simulink model "OFDM_Tx_HW_bk"  (R2020a)
settings: Solver=FixedStepDiscrete  StartTime=0.0  StopTime=inf  RelTol=1e-3
InitFcn:
  | % Set parameters
  | fs = 1e6;
  | 
  | % Load all required variables
  | load('variables/read_addr_data');
  | load('variables/read_addr_cp');
  | load('variables/read_addr_pream');
  | load('variables/read_addr_rx');
  | load('variables/pilot');
  | load('variables/sc_index');
  | load('variables/LTSfreq');
  | load('variables/STSfreq');
  | load('variables/LTSread');
  | load('variables/STSread');
  | 
  | run ./scripts/rfgen;
values from neighbouring files (symbols this model uses):
  interpolation_single = dsp.SampleRateConverter('InputSampleRate', 1e6,     'OutputSampleRate', 256e6,     'Bandwidth', 812.5e3,     'OutputRateTolerance', 0,     'StopbandAttenuation', 100)    [filter_design_1mhz.m]
undefined symbols (not defined in the file or in its folder): CIC_fine_Rx, Interpolate, lib_interpolatetx, lib_ofdmtx, LTSfreq, LTSread, OFDMTx, pilot, read_addr_cp, read_addr_data, read_addr_pream, STSfreq, STSread
libraries: hdlsllib x47, xbsIndex_r4 x22, simulink x19, dspsigops x5, dspmlti4 x3, lib_ofdmrx x1, lib_rfsignalgenerator x1, dsphdlxfrm x1, dspobslib x1
(part 1 of 2)
settings Model: Creator=njb13206  LastModifiedBy=david
settings OptimizationCC: BlockReduction=off  ConditionallyExecuteInputs=off  DefaultParameterBehavior=Inlined
settings DebuggingCC: AlgebraicLoopMsg=error  IntegerOverflowMsg=none  ParameterPrecisionLossMsg=none  IntegerSaturationMsg=none
settings HardwareCC: ProdBitPerPointer=32  ProdBitPerSizeT=32  ProdBitPerPtrDiffT=32  ProdLargestAtomicFloat=None  ProdIntDivRoundTo=Undefined  ProdEndianess=Unspecified  ProdWordSize=32  ProdHWDeviceType=ASIC/FPGA->ASIC/FPGA  TargetBitPerPointer=64  TargetBitPerSizeT=64  TargetBitPerPtrDiffT=64  TargetLongLongMode=on  TargetIntDivRoundTo=Zero  TargetEndianess=LittleEndian  TargetWordSize=64  TargetHWDeviceType=Custom Processor->MATLAB Host Computer  ProdEqTarget=off

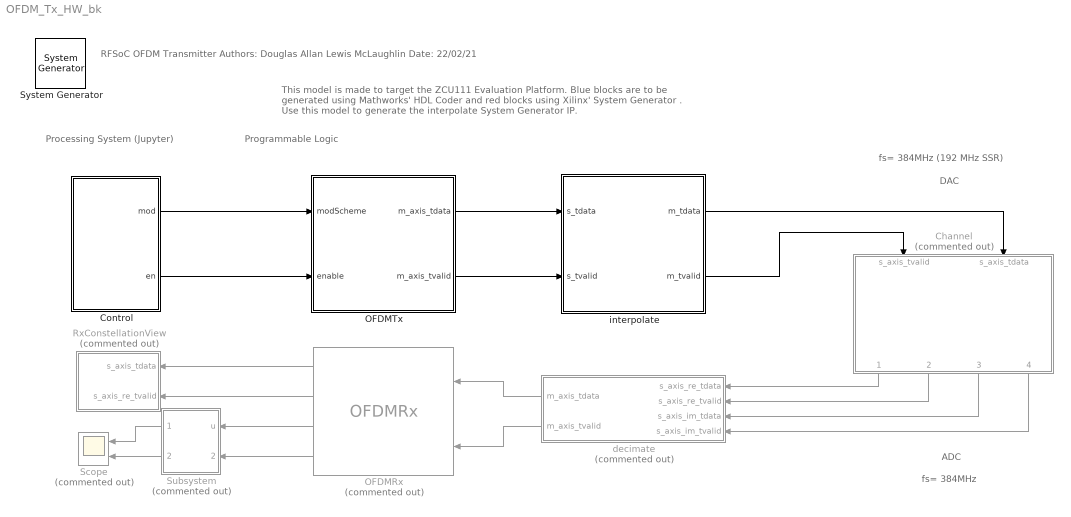
== system OFDM_Tx_HW_bk ==
  note: This model is made to target the ZCU111 Evaluation Platform. Blue blocks are to be generated using Mathworks' HDL Coder and red blocks using Xilinx' System Generator .
      |
      | Use this model to generate the interpolate System Generator IP.
  note: Programmable Logic
  note: Processing System (Jupyter)
  note: DAC
  note: fs= 384MHz (192 MHz SSR)
  note: ADC
  note: fs= 384MHz
  note: RFSoC OFDM Transmitter
      | Authors: Douglas Allan
      | Lewis McLaughlin
      | Date: 22/02/21
  " System Generator" : xbsIndex_r4/ System Generator  Tag=genX  xilinxfamily=zynquplusRFSOC  part=xczu28dr  speed=-2-e  package=ffvg1517  synthesis_tool=Vivado  clock_wrapper=Clock Enables  directory=./netlist  proj_type=Vivado  Synth_file=Vivado Synthesis Defaults  Impl_file=Vivado Implementation Defaults  testbench=off  simulink_period=1/256e6  sysclk_period=(1/256e6)*1e9  dcm_input_clock_period=10  incr_netlist=off  trim_vbits=Everywhere in SubSystem  dbl_ovrd=According to Block Masks  core_generation=According to Block Masks  run_coregen=off  deprecated_control=off  eval_field=0  block_type=sysgen
  Channel : Subsystem  Commented=on
  Control : Subsystem  mask{mod_mask=512QAM, en=on}
      mask prompts: mod_mask "Modulation"; en "Enable"
      mask init:
      | % RF Signal Generator
      | if strcmpi(get_param(gcb, 'mod_mask'), 'BPSK')
      |     mod = 0;
      | elseif strcmpi(get_param(gcb, 'mod_mask'), 'QPSK')
      |     mod = 1;
      | elseif strcmpi(get_param(gcb, 'mod_mask'), '8PSK')
      |     mod = 2;
      | elseif strcmpi(get_param(gcb, 'mod_mask'), '16QAM')
      |     mod = 3;
      | elseif strcmpi(get_param(gcb, 'mod_mask'), '32QAM')
      |     mod = 4;
      | elseif strcmpi(get_param(gcb, 'mod_mask'), '64QAM')
      |     mod = 5;
      | elseif strcmpi(get_param(gcb, 'mod_mask'), '128QAM')
      |     mod = 6;
      | elseif strcmpi(get_param(gcb, 'mod_mask'), '256QAM')
      |     mod = 7;
      | elseif strcmpi(get_param(gcb, 'mod_mask'), '512QAM')
      |     mod = 8;
      | elseif strcmpi(get_param(gcb, 'mod_mask'), '1024QAM')
      |     mod = 9;
      | end
      mask TypeOptions mod_mask: BPSK | QPSK | 8PSK | 16QAM | 32QAM | 64QAM | 128QAM | 256QAM | 512QAM | 1024QAM
      mask DialogControl DescGroupVar Prompt: RF Signal Generator
      mask DialogControl DescTextVar Prompt: Exposes parameters the user can control from Jupyter when running on the target.
      mask DialogControl Container3 Prompt: Control
  OFDMRx : lib_ofdmrx/OFDMRx  Commented=on  SystemSampleTime=-1  Latency=0  AutoFrameSizeCalculation=off
  OFDMTx : Subsystem  AncestorBlock=lib_ofdmtx/OFDMTx  TreatAsAtomicUnit=on
  RxConstellationView : Subsystem  Commented=on
  Scope : Scope  Commented=on  NumInputPorts=2
  Subsystem : Subsystem  Commented=on
  decimate : Subsystem  Commented=on
  interpolate : Subsystem  AncestorBlock=lib_interpolatetx/Interpolate
  wires:
  interpolate/1(m_tdata) -> Channel/2(s_axis_tdata)
  OFDMTx/1(m_axis_tdata) -> interpolate/1(s_tdata)
  OFDMTx/2(m_axis_tvalid) -> interpolate/2(s_tvalid)
  interpolate/2(m_tvalid) -> Channel/1(s_axis_tvalid)
  Channel/4(m_axis_im_tvalid) -> decimate/4(s_axis_im_tvalid)
  OFDMRx/1 -> RxConstellationView/1(s_axis_tdata)
  OFDMRx/2 -> RxConstellationView/2(s_axis_re_tvalid)
  Channel/1(m00_axis_re_tdata) -> decimate/1(s_axis_re_tdata)
  Channel/2(m_axis_re_tvalid) -> decimate/2(s_axis_re_tvalid)
  Channel/3(m01_axis_im_tdata) -> decimate/3(s_axis_im_tdata)
  decimate/2(m_axis_tvalid) -> OFDMRx/2
  decimate/1(m_axis_tdata) -> OFDMRx/1
  Control/1(mod) -> OFDMTx/1(modScheme)
  Control/2(en) -> OFDMTx/2(enable)
  OFDMRx/3 -> Subsystem/1(u)
  OFDMRx/4 -> Subsystem/2(tvalid)
  Subsystem/2(Out2) -> Scope/2
  Subsystem/1(Out1) -> Scope/1

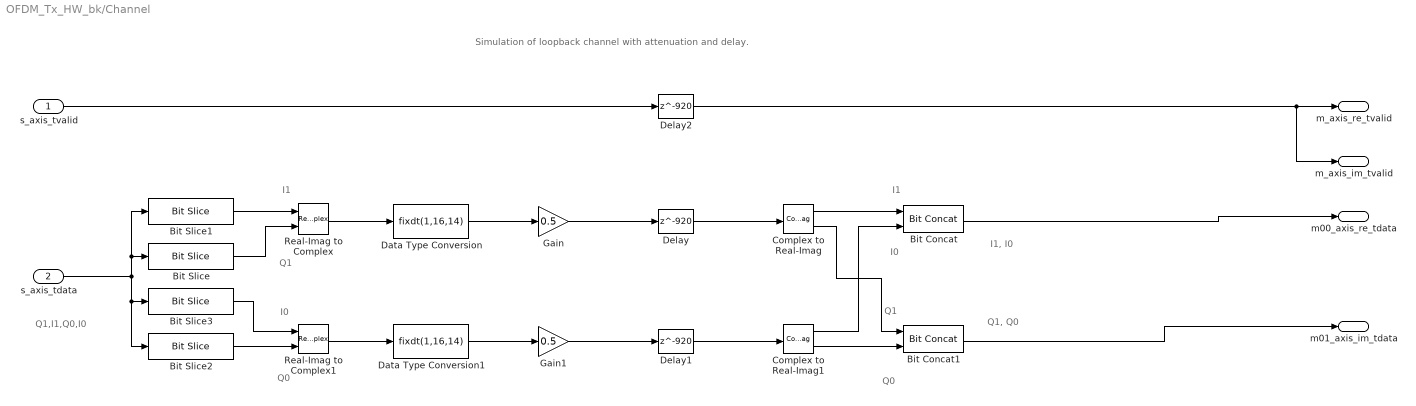
== system OFDM_Tx_HW_bk/Channel ==
  note: Q1, Q0
  note: I1, I0
  note: Q0
  note: I0
  note: Q1
  note: I1
  note: Q1,I1,Q0,I0
  note: Simulation of loopback channel with attenuation and delay.
  note: I1
  note: I0
  note: Q1
  note: Q0
  s_axis_tvalid : Inport
  s_axis_tdata : Inport  Port=2
  Bit Concat : hdlsllib/Logic and Bit Operations/Bit Concat  numInputs=2
  Bit Concat1 : hdlsllib/Logic and Bit Operations/Bit Concat  numInputs=2
  Bit Slice : hdlsllib/Logic and Bit Operations/Bit Slice  lidx=63  ridx=48
      settings: SourceProductBaseCode=SL
  Bit Slice1 : hdlsllib/Logic and Bit Operations/Bit Slice  lidx=47  ridx=32
      settings: SourceProductBaseCode=SL
  Bit Slice2 : hdlsllib/Logic and Bit Operations/Bit Slice  lidx=31  ridx=16
      settings: SourceProductBaseCode=SL
  Bit Slice3 : hdlsllib/Logic and Bit Operations/Bit Slice  lidx=15  ridx=0
      settings: SourceProductBaseCode=SL
  Complex to Real-Imag : ComplexToRealImag
  Complex to Real-Imag1 : ComplexToRealImag
  Data Type Conversion : DataTypeConversion  OutDataTypeStr=fixdt(1,16,14)  ConvertRealWorld=Stored Integer (SI)
  Data Type Conversion1 : DataTypeConversion  OutDataTypeStr=fixdt(1,16,14)  ConvertRealWorld=Stored Integer (SI)
  Delay : Delay  DelayLength=920
  Delay1 : Delay  DelayLength=920
  Delay2 : Delay  DelayLength=920
  Gain : Gain  Gain=0.5  ParamDataTypeStr=double  OutDataTypeStr=fixdt(1,16,14)
  Gain1 : Gain  Gain=0.5  ParamDataTypeStr=double  OutDataTypeStr=fixdt(1,16,14)
  Real-Imag to Complex : RealImagToComplex
  Real-Imag to Complex1 : RealImagToComplex
  m00_axis_re_tdata : Outport  VectorParamsAs1DForOutWhenUnconnected=off
  m_axis_re_tvalid : Outport  Port=2  VectorParamsAs1DForOutWhenUnconnected=off
  m01_axis_im_tdata : Outport  Port=3  VectorParamsAs1DForOutWhenUnconnected=off
  m_axis_im_tvalid : Outport  Port=4  VectorParamsAs1DForOutWhenUnconnected=off
  wires:
  Gain/1 -> Delay/1
  s_axis_tvalid/1 -> Delay2/1
  Delay/1 -> Complex to Real-Imag/1
  s_axis_tdata/1 -> Bit Slice1/1, Bit Slice/1, Bit Slice2/1, Bit Slice3/1
  Delay1/1 -> Complex to Real-Imag1/1
  Gain1/1 -> Delay1/1
  Bit Concat/1 -> m00_axis_re_tdata/1
  Bit Concat1/1 -> m01_axis_im_tdata/1
  Bit Slice/1 -> Real-Imag to Complex/2
  Bit Slice1/1 -> Real-Imag to Complex/1
  Bit Slice2/1 -> Real-Imag to Complex1/2
  Bit Slice3/1 -> Real-Imag to Complex1/1
  Real-Imag to Complex/1 -> Data Type Conversion/1
  Real-Imag to Complex1/1 -> Data Type Conversion1/1
  Complex to Real-Imag1/1 -> Bit Concat/2
  Complex to Real-Imag/1 -> Bit Concat/1
  Complex to Real-Imag1/2 -> Bit Concat1/2
  Complex to Real-Imag/2 -> Bit Concat1/1
  Data Type Conversion/1 -> Gain/1
  Data Type Conversion1/1 -> Gain1/1
  Delay2/1 -> m_axis_im_tvalid/1, m_axis_re_tvalid/1

== system OFDM_Tx_HW_bk/Control ==
  Constant2 : Constant  Value=en  OutDataTypeStr=boolean  SampleTime=1/(fs)
  Constant7 : Constant  Value=mod  VectorParams1D=off  OutDataTypeStr=uint32  SampleTime=1/(fs)
  Delay : Delay  DelayLength=randi(10)
  Delay3 : Delay  DelayLength=randi(10)
  mod : Outport  VectorParamsAs1DForOutWhenUnconnected=off
  en : Outport  Port=2  VectorParamsAs1DForOutWhenUnconnected=off
  wires:
  Constant2/1 -> Delay3/1
  Constant7/1 -> Delay/1
  Delay/1 -> mod/1
  Delay3/1 -> en/1

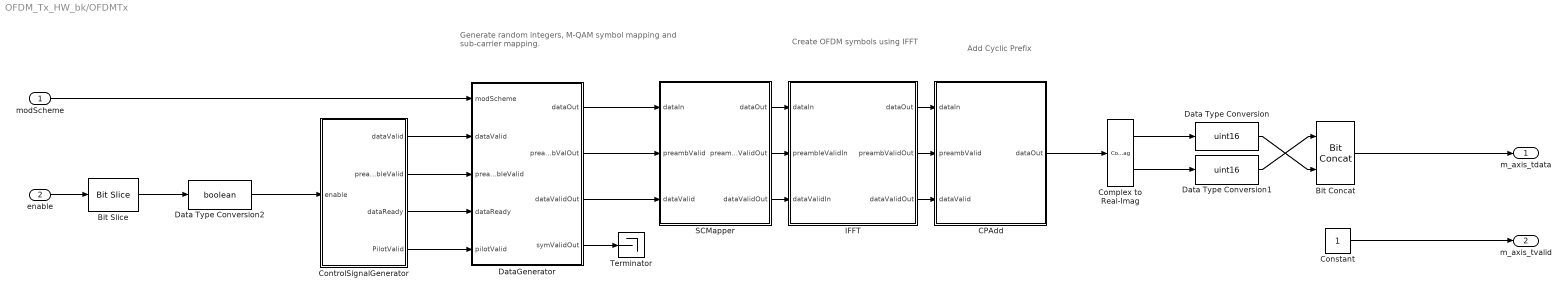
== system OFDM_Tx_HW_bk/OFDMTx ==
  note: Generate random integers, M-QAM symbol mapping and sub-carrier
      | mapping.
  note: Add Cyclic Prefix
  note: Create OFDM symbols using
      | IFFT
  modScheme : Inport
  enable : Inport  Port=2
  Bit Concat : hdlsllib/Logic and Bit Operations/Bit Concat  numInputs=2
  Bit Slice : hdlsllib/Logic and Bit Operations/Bit Slice  lidx=0  ridx=0
      settings: SourceProductBaseCode=SL
  CPAdd : Subsystem
  Complex to Real-Imag : ComplexToRealImag
  Constant : Constant  OutDataTypeStr=boolean  SampleTime=1/fs
  ControlSignalGenerator : Subsystem
  Data Type Conversion : DataTypeConversion  OutDataTypeStr=uint16  ConvertRealWorld=Stored Integer (SI)
  Data Type Conversion1 : DataTypeConversion  OutDataTypeStr=uint16  ConvertRealWorld=Stored Integer (SI)
  Data Type Conversion2 : DataTypeConversion  OutDataTypeStr=boolean  ConvertRealWorld=Stored Integer (SI)
  DataGenerator : Subsystem
  IFFT : Subsystem
  SCMapper : Subsystem
  Terminator : Terminator
  m_axis_tdata : Outport  VectorParamsAs1DForOutWhenUnconnected=off
  m_axis_tvalid : Outport  Port=2  VectorParamsAs1DForOutWhenUnconnected=off
  wires:
  Bit Slice/1 -> Data Type Conversion2/1
  enable/1 -> Bit Slice/1
  Data Type Conversion/1 -> Bit Concat/2
  Data Type Conversion1/1 -> Bit Concat/1
  Complex to Real-Imag/2 -> Data Type Conversion1/1
  Complex to Real-Imag/1 -> Data Type Conversion/1
  Bit Concat/1 -> m_axis_tdata/1
  modScheme/1 -> DataGenerator/1(modScheme)
  DataGenerator/1(dataOut) -> SCMapper/1(dataIn)
  DataGenerator/2(preambValOut) -> SCMapper/2(preambValid)
  DataGenerator/3(dataValidOut) -> SCMapper/3(dataValid)
  SCMapper/1(dataOut) -> IFFT/1(dataIn)
  SCMapper/2(preambValidOut) -> IFFT/2(preambleValidIn)
  SCMapper/3(dataValidOut) -> IFFT/3("dataValidIn ")
  IFFT/1(dataOut) -> CPAdd/1(dataIn)
  IFFT/2(preambValidOut) -> CPAdd/2(preambValid)
  IFFT/3(dataValidOut) -> CPAdd/3(dataValid)
  CPAdd/1(dataOut) -> Complex to Real-Imag/1
  ControlSignalGenerator/1(dataValid) -> DataGenerator/2(dataValid)
  ControlSignalGenerator/2(preambleValid) -> DataGenerator/3(preambleValid)
  ControlSignalGenerator/3(dataReady) -> DataGenerator/4(dataReady)
  ControlSignalGenerator/4(PilotValid) -> DataGenerator/5(pilotValid)
  Data Type Conversion2/1 -> ControlSignalGenerator/1(enable)
  Constant/1 -> m_axis_tvalid/1
  DataGenerator/4(symValidOut) -> Terminator/1

== system OFDM_Tx_HW_bk/RxConstellationView ==
  s_axis_tdata : Inport
  s_axis_re_tvalid : Inport  Port=2
  Bit Slice : hdlsllib/Logic and Bit Operations/Bit Slice  lidx=15  ridx=0
      settings: SourceProductBaseCode=SL
  Bit Slice1 : hdlsllib/Logic and Bit Operations/Bit Slice  lidx=31  ridx=16
      settings: SourceProductBaseCode=SL
  Constant : Constant  Value=NaN + 1i*NaN  OutDataTypeStr=double  SampleTime=-1
  Constellation Diagram : ConstellationDiagram
  Data Type Conversion : DataTypeConversion  OutDataTypeStr=fixdt(1,16,14)  ConvertRealWorld=Stored Integer (SI)
  Real-Imag to Complex : RealImagToComplex
  Switch : Switch  Criteria=u2 ~= 0
  wires:
  Switch/1 -> Constellation Diagram/1
  Constant/1 -> Switch/3
  s_axis_re_tvalid/1 -> Switch/2
  Real-Imag to Complex/1 -> Data Type Conversion/1
  Bit Slice/1 -> Real-Imag to Complex/1
  s_axis_tdata/1 -> Bit Slice1/1, Bit Slice/1
  Bit Slice1/1 -> Real-Imag to Complex/2
  Data Type Conversion/1 -> Switch/1

== system OFDM_Tx_HW_bk/Subsystem ==
  u : Inport
  tvalid : Inport  Port=2
  Abs : Abs
  Bit Slice : hdlsllib/Logic and Bit Operations/Bit Slice  lidx=15  ridx=0
      settings: SourceProductBaseCode=SL
  Bit Slice1 : hdlsllib/Logic and Bit Operations/Bit Slice  lidx=31  ridx=16
      settings: SourceProductBaseCode=SL
  Data Type Conversion1 : DataTypeConversion  OutDataTypeStr=fixdt(1,16,14)  ConvertRealWorld=Stored Integer (SI)
  Data Type Conversion2 : DataTypeConversion  OutDataTypeStr=double
  Real-Imag to Complex : RealImagToComplex
  Out1 : Outport
  Out2 : Outport  Port=2
  wires:
  Bit Slice/1 -> Real-Imag to Complex/1
  u/1 -> Bit Slice/1, Bit Slice1/1
  Real-Imag to Complex/1 -> Data Type Conversion1/1
  Bit Slice1/1 -> Real-Imag to Complex/2
  Abs/1 -> Out1/1
  Data Type Conversion1/1 -> Data Type Conversion2/1
  Data Type Conversion2/1 -> Abs/1
  tvalid/1 -> Out2/1

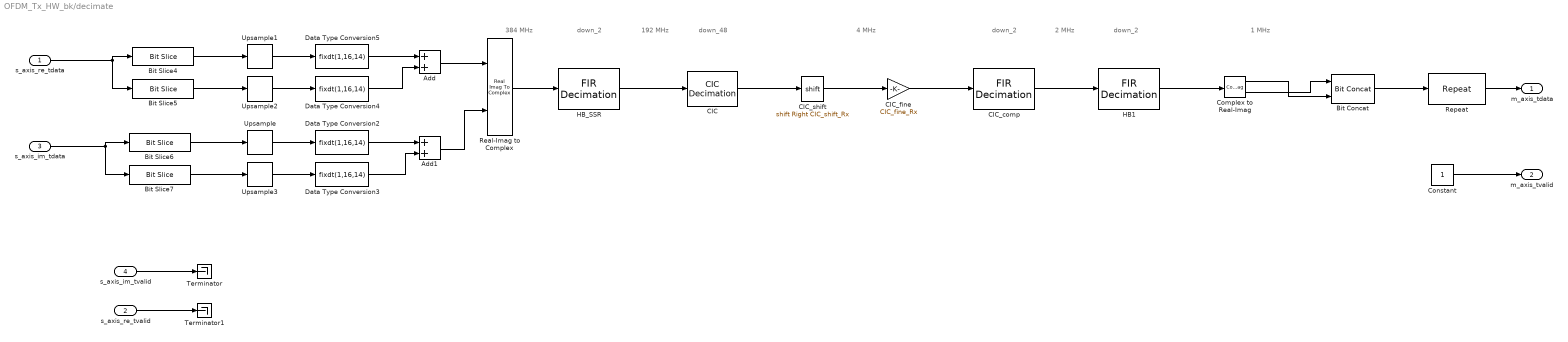
== system OFDM_Tx_HW_bk/decimate ==
  note: down_2
  note: 2 MHz
  note: 4 MHz
  note: 192 MHz
  note: 384 MHz
  note: 1 MHz
  note: down_48
  note: down_2
  note: down_2
  s_axis_re_tdata : Inport
  s_axis_re_tvalid : Inport  Port=2
  s_axis_im_tdata : Inport  Port=3
  s_axis_im_tvalid : Inport  Port=4
  Add : Sum  OutDataTypeStr=fixdt(1,16,14)
  Add1 : Sum  OutDataTypeStr=fixdt(1,16,14)
  Bit Concat : hdlsllib/Logic and Bit Operations/Bit Concat  numInputs=2
  Bit Slice4 : hdlsllib/Logic and Bit Operations/Bit Slice  lidx=15  ridx=0
      settings: SourceProductBaseCode=SL
  Bit Slice5 : hdlsllib/Logic and Bit Operations/Bit Slice  lidx=31  ridx=16
      settings: SourceProductBaseCode=SL
  Bit Slice6 : hdlsllib/Logic and Bit Operations/Bit Slice  lidx=15  ridx=0
      settings: SourceProductBaseCode=SL
  Bit Slice7 : hdlsllib/Logic and Bit Operations/Bit Slice  lidx=31  ridx=16
      settings: SourceProductBaseCode=SL
  CIC : dspobslib/CIC Decimation  filtFrom=Multirate object in workspace  filtobj=CIC_Rx  ftype=Decimator  R=2  M=1  N=2  filterInternals=Full precision  BPS=[16 16 16 16]  FLPS=0  outputWordLength=32  outputFracLength=0  launchFVT=off  framing=Maintain input frame rate  RateOptions=Allow multirate processing
      settings: SourceProductBaseCode=DS
  CIC_comp : dspmlti4/FIR Decimation  FilterSource=Dialog parameters  h=WComp_Rx.Numerator  D=2  filtStruct=Direct form  FilterObject=FDECIM  framing=Allow multirate processing  inputOffset=0  outputBufInitCond=0  roundingMode=Floor  overflowMode=off  firstCoeffMode=Binary point scaling  firstCoeffWordLength=16  firstCoeffFracLength=15  firstCoeffDataTypeStr=fixdt(1,16,15)  firstCoeffMin=[]  firstCoeffMax=[]  firstCoeffLastDataTypeStr=fixdt(1,16,15)  outputMode=Binary point scaling  outputWordLength=16  outputFracLength=14  outputDataTypeStr=fixdt(1,16,14)  outputMin=[]  outputMax=[]  outputLastDataTypeStr=fixdt(1,16,14)
  CIC_fine : Gain  Gain=CIC_fine_Rx  OutDataTypeStr=fixdt(1,16,14)
  CIC_shift : ArithShift  BitShiftNumber=CIC_shift_Rx  BitShiftDirection=Right
  Complex to Real-Imag : ComplexToRealImag
  Constant : Constant  OutDataTypeStr=boolean  SampleTime=1/(fs*12)
  Data Type Conversion{2..5} (4 alike) : DataTypeConversion  OutDataTypeStr=fixdt(1,16,14)  ConvertRealWorld=Stored Integer (SI)
  HB1 : dspmlti4/FIR Decimation  FilterSource=Dialog parameters  h=W_HB.Numerator  D=2  filtStruct=Direct form  FilterObject=FDECIM  framing=Allow multirate processing  inputOffset=0  outputBufInitCond=0  roundingMode=Floor  overflowMode=off  firstCoeffMode=Binary point scaling  firstCoeffWordLength=16  firstCoeffFracLength=15  firstCoeffDataTypeStr=fixdt(1,16,15)  firstCoeffMin=[]  firstCoeffMax=[]  firstCoeffLastDataTypeStr=fixdt(1,16,15)  outputMode=Binary point scaling  outputWordLength=16  outputFracLength=14  outputDataTypeStr=fixdt(1,16,14)  outputMin=[]  outputMax=[]  outputLastDataTypeStr=fixdt(1,16,14)
  HB_SSR : dspmlti4/FIR Decimation  FilterSource=Dialog parameters  h=W_HB.Numerator  D=2  filtStruct=Direct form  FilterObject=FDECIM  framing=Allow multirate processing  inputOffset=0  outputBufInitCond=0  roundingMode=Floor  overflowMode=off  firstCoeffMode=Binary point scaling  firstCoeffWordLength=16  firstCoeffFracLength=15  firstCoeffDataTypeStr=fixdt(1,16,15)  firstCoeffMin=[]  firstCoeffMax=[]  firstCoeffLastDataTypeStr=fixdt(1,16,15)  outputMode=Binary point scaling  outputWordLength=16  outputFracLength=14  outputDataTypeStr=fixdt(1,16,14)  outputMin=[]  outputMax=[]  outputLastDataTypeStr=fixdt(1,16,14)
  Real-Imag to Complex : RealImagToComplex
  Repeat : dspsigops/Repeat  N=12  InputProcessing=Columns as channels (frame based)  RateOptions=Allow multirate processing  ic=0  mode=Unused parameter value
  Terminator : Terminator
  Terminator1 : Terminator
  Upsample : dspsigops/Upsample  N=2  phase=0  RateOptions=Allow multirate processing  ic=0  mode=Unused parameter value
  Upsample1 : dspsigops/Upsample  N=2  phase=0  RateOptions=Allow multirate processing  ic=0  mode=Unused parameter value
  Upsample2 : dspsigops/Upsample  N=2  phase=1  RateOptions=Allow multirate processing  ic=0  mode=Unused parameter value
  Upsample3 : dspsigops/Upsample  N=2  phase=1  RateOptions=Allow multirate processing  ic=0  mode=Unused parameter value
  m_axis_tdata : Outport
  m_axis_tvalid : Outport  Port=2
  wires:
  CIC_comp/1 -> HB1/1
  CIC_shift/1 -> CIC_fine/1
  HB_SSR/1 -> CIC/1
  CIC/1 -> CIC_shift/1
  CIC_fine/1 -> CIC_comp/1
  HB1/1 -> Complex to Real-Imag/1
  Real-Imag to Complex/1 -> HB_SSR/1
  s_axis_im_tvalid/1 -> Terminator/1
  s_axis_re_tvalid/1 -> Terminator1/1
  Repeat/1 -> m_axis_tdata/1
  Data Type Conversion3/1 -> Add1/2
  Data Type Conversion5/1 -> Add/1
  Upsample2/1 -> Data Type Conversion4/1
  Upsample3/1 -> Data Type Conversion3/1
  Data Type Conversion4/1 -> Add/2
  Bit Slice7/1 -> Upsample3/1
  Bit Slice6/1 -> Upsample/1
  Upsample/1 -> Data Type Conversion2/1
  Add/1 -> Real-Imag to Complex/1
  Bit Slice5/1 -> Upsample2/1
  Data Type Conversion2/1 -> Add1/1
  s_axis_re_tdata/1 -> Bit Slice4/1, Bit Slice5/1
  Add1/1 -> Real-Imag to Complex/2
  s_axis_im_tdata/1 -> Bit Slice6/1, Bit Slice7/1
  Upsample1/1 -> Data Type Conversion5/1
  Bit Slice4/1 -> Upsample1/1
  Complex to Real-Imag/1 -> Bit Concat/2
  Complex to Real-Imag/2 -> Bit Concat/1
  Bit Concat/1 -> Repeat/1
  Constant/1 -> m_axis_tvalid/1

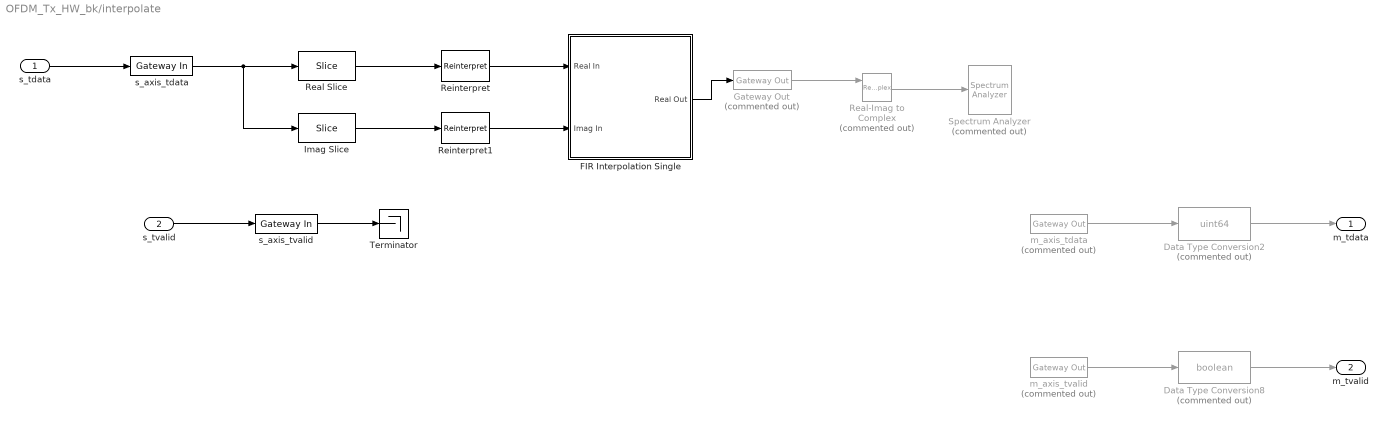
== system OFDM_Tx_HW_bk/interpolate ==
  s_tdata : Inport
  s_tvalid : Inport  Port=2
  Data Type Conversion2 : DataTypeConversion  Commented=on  OutDataTypeStr=uint64  ConvertRealWorld=Stored Integer (SI)
  Data Type Conversion8 : DataTypeConversion  Commented=on  OutDataTypeStr=boolean  ConvertRealWorld=Stored Integer (SI)
  FIR Interpolation Single : Subsystem
  Gateway Out : xbsIndex_r4/Gateway Out  Commented=on  inherit_from_input=on  hdl_port=off  rows=1  columns=1  UseAsDAC=off  DACChannel='1'  interface=None  automatic_assignment=on  address_offset=hex2dec('00')  intf_name=''  intf_description=''  timing_constraint=None  locs_specified=off  LOCs={}  io_standard={}  block_type=gatewayout
  Imag Slice : xbsIndex_r4/Slice  nbits=1  boolean_output=off  mode=Two Bit Locations  bit1=31  base1=LSB of Input  bit0=16  base0=LSB of Input  dbl_ovrd=off  block_type=slice
  Real Slice : xbsIndex_r4/Slice  nbits=1  boolean_output=off  mode=Two Bit Locations  bit1=15  base1=LSB of Input  bit0=0  base0=LSB of Input  dbl_ovrd=off  block_type=slice
  Real-Imag to Complex : RealImagToComplex  Commented=on
  Reinterpret : xbsIndex_r4/Reinterpret  force_arith_type=on  arith_type="Signed  (2's comp)"  force_bin_pt=on  bin_pt=15  block_type=reinterpret
  Reinterpret1 : xbsIndex_r4/Reinterpret  force_arith_type=on  arith_type="Signed  (2's comp)"  force_bin_pt=on  bin_pt=15  block_type=reinterpret
  Spectrum Analyzer : SpectrumAnalyzer  Commented=on
  Terminator : Terminator
  m_axis_tdata : xbsIndex_r4/Gateway Out  Commented=on  inherit_from_input=on  hdl_port=on  rows=1  columns=1  UseAsDAC=off  DACChannel='1'  interface=None  automatic_assignment=on  address_offset=hex2dec('00')  intf_name=''  intf_description=''  timing_constraint=None  locs_specified=off  LOCs={}  io_standard={}  block_type=gatewayout
  m_axis_tvalid : xbsIndex_r4/Gateway Out  Commented=on  inherit_from_input=on  hdl_port=on  rows=1  columns=1  UseAsDAC=off  DACChannel='1'  interface=None  automatic_assignment=on  address_offset=hex2dec('00')  intf_name=''  intf_description=''  timing_constraint=None  locs_specified=off  LOCs={}  io_standard={}  block_type=gatewayout
      settings: infoedit=The Vector Real Gateway out block converts Xilinx fixed-point or floating-point type vector inputs into vector ouputs of type Simulink integer, single, double, or fixed-point.<br><br>Hardware notes: In hardware these blocks become top level output ports or are discarded, depending on how they are configured.
  s_axis_tdata : xbsIndex_r4/Gateway In  gui_display_data_type=Fixed-point  arith_type=Unsigned  n_bits=32  bin_pt=0  preci_type=Single  exp_width=8  frac_width=24  rows=1  columns=1  quantization="Round  (unbiased: +/- Inf)"  overflow=Saturate  period=1/(fs)  UseAsADC=off  ADCChannel='1'  interface=None  automatic_assignment=on  address_offset=hex2dec('00')  intf_name=''  intf_description=''  default_value=0  timing_constraint=None  locs_specified=off  LOCs={}  io_standard={}  inherit_from_input=off  hdl_port=on  dbl_ovrd=off  block_type=gatewayin
  s_axis_tvalid : xbsIndex_r4/Gateway In  gui_display_data_type=Boolean  arith_type=Boolean  n_bits=32  bin_pt=0  preci_type=Single  exp_width=8  frac_width=24  rows=1  columns=1  quantization="Round  (unbiased: +/- Inf)"  overflow=Saturate  period=1/(fs)  UseAsADC=off  ADCChannel='1'  interface=None  automatic_assignment=on  address_offset=hex2dec('00')  intf_name=''  intf_description=''  default_value=0  timing_constraint=None  locs_specified=off  LOCs={}  io_standard={}  inherit_from_input=off  hdl_port=on  dbl_ovrd=off  block_type=gatewayin
  m_tdata : Outport
  m_tvalid : Outport  Port=2
  wires:
  Data Type Conversion8/1 -> m_tvalid/1
  s_tvalid/1 -> s_axis_tvalid/1
  Data Type Conversion2/1 -> m_tdata/1
  m_axis_tdata/1 -> Data Type Conversion2/1
  m_axis_tvalid/1 -> Data Type Conversion8/1
  s_tdata/1 -> s_axis_tdata/1
  s_axis_tvalid/1 -> Terminator/1
  Gateway Out/1 -> Real-Imag to Complex/1
  Real-Imag to Complex/1 -> Spectrum Analyzer/1
  s_axis_tdata/1 -> Imag Slice/1, Real Slice/1
  FIR Interpolation Single/1(Real Out) -> Gateway Out/1
  Real Slice/1 -> Reinterpret/1
  Imag Slice/1 -> Reinterpret1/1
  Reinterpret/1 -> FIR Interpolation Single/1(Real In)
  Reinterpret1/1 -> FIR Interpolation Single/2(Imag In)

== system OFDM_Tx_HW_bk/OFDMTx/CPAdd ==
  dataIn : Inport
  preambValid : Inport  Port=2
  dataValid : Inport  Port=3
  DataExtend : Subsystem
  LTFExtend : Subsystem
  Mux2 : MATLAB Function  TreatAsAtomicUnit=on
  STFExtend : Subsystem
  dataOut : Outport  VectorParamsAs1DForOutWhenUnconnected=off
  wires:
  preambValid/1 -> LTFExtend/2(preambVal), STFExtend/2(preambVal)
  dataIn/1 -> DataExtend/1(dataIn), LTFExtend/1(data), STFExtend/1(data)
  STFExtend/1(STFExtendOut) -> Mux2/1(sts)
  STFExtend/2(STFValidOut) -> Mux2/2(stsval)
  LTFExtend/1(LTFExtendOut) -> Mux2/3(lts)
  LTFExtend/2(LTFValidOut) -> Mux2/4(ltsval)
  DataExtend/1(dataOut) -> Mux2/5(data)
  DataExtend/2(dataValidOut) -> Mux2/6(dataval)
  Mux2/1(dataOut) -> dataOut/1
  dataValid/1 -> DataExtend/2(dataValid)

== system OFDM_Tx_HW_bk/OFDMTx/ControlSignalGenerator ==
  enable : Inport
  PreamValidGen : Subsystem
  dataReadyGen : Subsystem
  dataValidGen : Subsystem
  pilotValidGen : Subsystem
  dataValid : Outport
  preambleValid : Outport  Port=2
  dataReady : Outport  Port=3
  PilotValid : Outport  Port=4
  wires:
  enable/1 -> dataValidGen/2(enable), PreamValidGen/1(enable)
  dataReadyGen/1(y) -> dataReady/1
  pilotValidGen/1(y) -> PilotValid/1
  PreamValidGen/1(y) -> preambleValid/1, dataValidGen/1(y)
  dataValidGen/1(valOut) -> pilotValidGen/1(enb), dataReadyGen/1(enb), dataValid/1

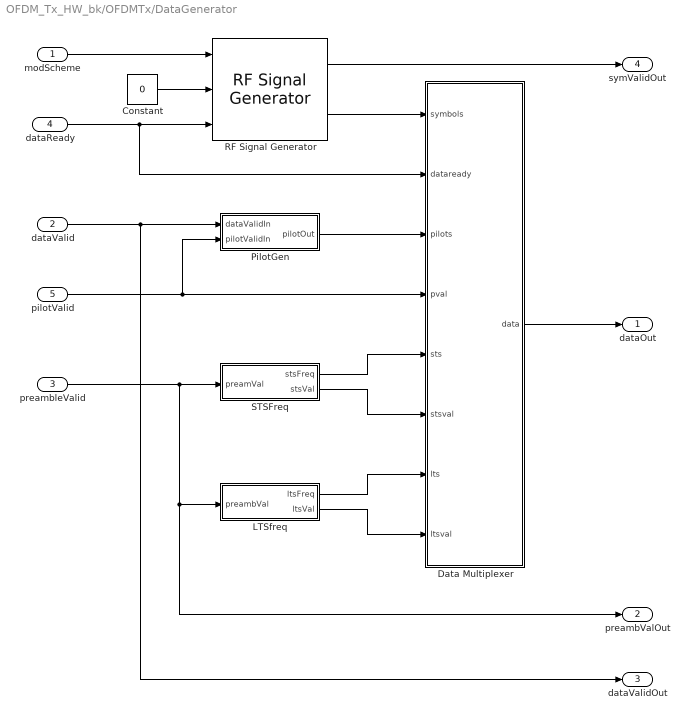
== system OFDM_Tx_HW_bk/OFDMTx/DataGenerator ==
  modScheme : Inport
  dataValid : Inport  Port=2
  preambleValid : Inport  Port=3
  dataReady : Inport  Port=4
  pilotValid : Inport  Port=5
  Constant : Constant  Value=0  OutDataTypeStr=boolean  SampleTime=1/fs
  Data Multiplexer : MATLAB Function  TreatAsAtomicUnit=on
  LTSfreq : Subsystem
  PilotGen : Subsystem
  RF Signal Generator : lib_rfsignalgenerator/RF Signal Generator  SystemSampleTime=-1  Latency=0  AutoFrameSizeCalculation=off
  STSFreq : Subsystem
  dataOut : Outport  VectorParamsAs1DForOutWhenUnconnected=off
  preambValOut : Outport  Port=2  VectorParamsAs1DForOutWhenUnconnected=off
  dataValidOut : Outport  Port=3  VectorParamsAs1DForOutWhenUnconnected=off
  symValidOut : Outport  Port=4  VectorParamsAs1DForOutWhenUnconnected=off
  wires:
  dataValid/1 -> PilotGen/1(dataValidIn), dataValidOut/1
  preambleValid/1 -> STSFreq/1(preamVal), LTSfreq/1(preambVal), preambValOut/1
  LTSfreq/2(ltsVal) -> Data Multiplexer/8(ltsval)
  LTSfreq/1(ltsFreq) -> Data Multiplexer/7(lts)
  STSFreq/2(stsVal) -> Data Multiplexer/6(stsval)
  STSFreq/1(stsFreq) -> Data Multiplexer/5(sts)
  pilotValid/1 -> PilotGen/2(pilotValidIn), Data Multiplexer/4(pval)
  PilotGen/1(pilotOut) -> Data Multiplexer/3(pilots)
  RF Signal Generator/2 -> Data Multiplexer/1(symbols)
  Data Multiplexer/1(data) -> dataOut/1
  modScheme/1 -> RF Signal Generator/1
  RF Signal Generator/1 -> symValidOut/1
  Constant/1 -> RF Signal Generator/2
  dataReady/1 -> RF Signal Generator/3, Data Multiplexer/2(dataready)

== system OFDM_Tx_HW_bk/OFDMTx/IFFT ==
  dataIn : Inport
  preambleValidIn : Inport  Port=2
  "dataValidIn " : Inport  Port=3
  Delay : Delay  DelayLength=173  InitialCondition=0  UseCircularBuffer=on
  Delay1 : Delay  DelayLength=173  InitialCondition=0  UseCircularBuffer=on
  IFFT HDL Optimized : dsphdlxfrm/IFFT HDL Optimized  FFTLength=64  Architecture=Streaming Radix 2^2  ComplexMultiplication=Use 3 multipliers and 5 adders  BitReversedOutput=off  BitReversedInput=off  Normalize=on  SimulateUsing=Code generation  RoundingMethod=Floor  ResetInputPort=off  StartOutputPort=off  EndOutputPort=off
      settings: SourceProductBaseCode=DS
  IFFTValid : Subsystem
  Terminator : Terminator
  dataOut : Outport  VectorParamsAs1DForOutWhenUnconnected=off
  preambValidOut : Outport  Port=2  VectorParamsAs1DForOutWhenUnconnected=off
  dataValidOut : Outport  Port=3  VectorParamsAs1DForOutWhenUnconnected=off
  wires:
  dataIn/1 -> IFFT HDL Optimized/1
  IFFT HDL Optimized/2 -> Terminator/1
  "dataValidIn "/1 -> IFFTValid/2(dataValid), Delay1/1
  IFFTValid/1(ifftValid) -> IFFT HDL Optimized/2
  preambleValidIn/1 -> IFFTValid/1(preambleValid), Delay/1
  Delay/1 -> preambValidOut/1
  Delay1/1 -> dataValidOut/1
  IFFT HDL Optimized/1 -> dataOut/1

== system OFDM_Tx_HW_bk/OFDMTx/SCMapper ==
  dataIn : Inport
  preambValid : Inport  Port=2
  dataValid : Inport  Port=3
  DataMapper : Subsystem
  Mux2 : MATLAB Function  TreatAsAtomicUnit=on
  PremableMapper : Subsystem
  dataOut : Outport  VectorParamsAs1DForOutWhenUnconnected=off
  preambValidOut : Outport  Port=2  VectorParamsAs1DForOutWhenUnconnected=off
  dataValidOut : Outport  Port=3  VectorParamsAs1DForOutWhenUnconnected=off
  wires:
  PremableMapper/1(preambleShiftOut) -> Mux2/1(preamb)
  PremableMapper/2(preambValOut) -> preambValidOut/1, Mux2/2(preambVal)
  DataMapper/1(dataOut) -> Mux2/3(data)
  DataMapper/2(dataValidOut) -> dataValidOut/1, Mux2/4(dataVal)
  dataIn/1 -> DataMapper/1(dataIn), PremableMapper/1(data)
  preambValid/1 -> PremableMapper/2(preambVal)
  dataValid/1 -> DataMapper/2(dataValid)
  Mux2/1(dataOut) -> dataOut/1

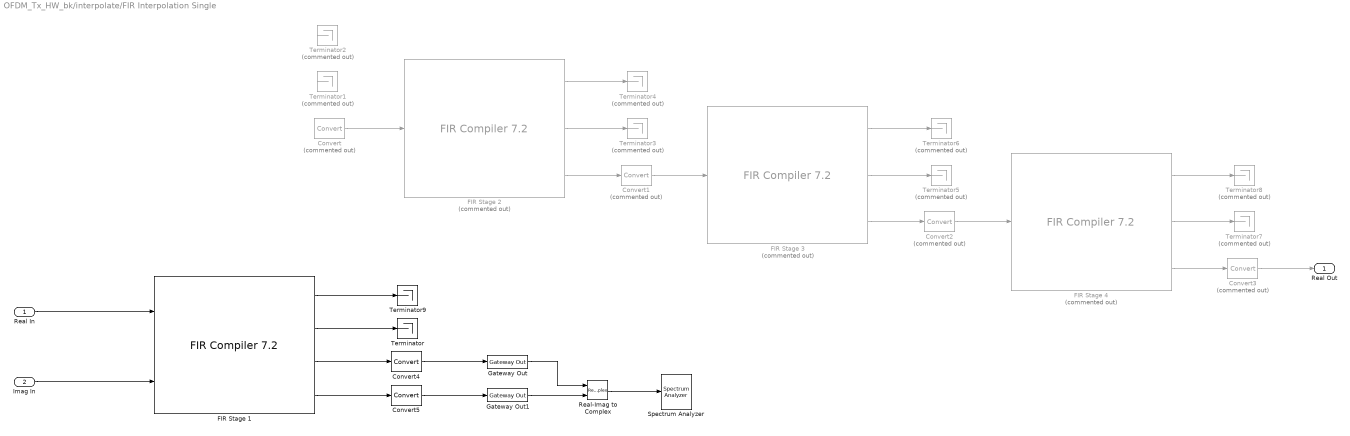
== system OFDM_Tx_HW_bk/interpolate/FIR Interpolation Single ==
  Real In : Inport
  Imag In : Inport  Port=2
  Convert{,1..3} (4 alike) : xbsIndex_r4/Convert  Commented=on  gui_display_data_type=Fixed-point  arith_type="Signed  (2's comp)"  n_bits=16  bin_pt=15  float_type=Single  exp_bits=8  fraction_bits=24  quantization="Round  (unbiased: +/- Inf)"  overflow=Saturate  en=off  latency=0  pipeline=off  dbl_ovrd=off  block_type=convert
  Convert4 : xbsIndex_r4/Convert  gui_display_data_type=Fixed-point  arith_type="Signed  (2's comp)"  n_bits=16  bin_pt=15  float_type=Single  exp_bits=8  fraction_bits=24  quantization="Round  (unbiased: +/- Inf)"  overflow=Saturate  en=off  latency=0  pipeline=off  dbl_ovrd=off  block_type=convert
  Convert5 : xbsIndex_r4/Convert  gui_display_data_type=Fixed-point  arith_type="Signed  (2's comp)"  n_bits=16  bin_pt=15  float_type=Single  exp_bits=8  fraction_bits=24  quantization="Round  (unbiased: +/- Inf)"  overflow=Saturate  en=off  latency=0  pipeline=off  dbl_ovrd=off  block_type=convert
  FIR Stage 1 : xbsIndex_r4/FIR Compiler 7.2   coefficientvector=interpolation_single.getFilters.Stage1.Numerator/2  coefficient_sets=1  coefficient_reload=off  filter_type=Interpolation  rate_change_type=Integer  interpolation_rate=2  decimation_rate=1  zero_pack_factor=1  channel_sequence=Basic  number_channels=1  pattern_list='P4-0,P4-1,P4-2,P4-3,P4-4'  number_paths=2  ratespecification=Maximum_Possible  sampleperiod=12  hardwareoversamplingrate=1  coefficient_sign=Signed  quantization=Quantize_Only  coefficient_width=16  bestprecision=on  coefficient_fractional_bits=15  coefficient_structure=Inferred  output_rounding_mode=Full_Precision  output_width=32  filter_architecture=Systolic_Multiply_Accumulate  optimization_goal=Area  optimization_list='None'  data_buffer_type=Automatic  coefficient_buffer_type=Automatic  input_buffer_type=Automatic  output_buffer_type=Automatic  preference_for_other_storage=Automatic  multi_column_support=Automatic  columnconfig='9'  inter_column_pipe_length=4  data_has_tlast=Not_Required  m_data_has_tready=off  s_data_has_fifo=off  s_data_has_tuser=Not_Required  m_data_has_tuser=Not_Required  s_config_sync_mode=On_Vector  s_config_method=Single  num_reload_slots=1  has_aclken=off  has_aresetn=off  infoeditControl=ARESETn must be asserted for a minimum of 2 cycles  reset_data_vector=on  trim_axipin_name=on  simulation_type=hybrid_sim  simulation_model=sysgen:xfirv7_2_cmodel  data_path_portlist={ 's_axis_data_tdata', 'm_axis_data_tdata' }  passband_min=0.0  passband_max=0.5  stopband_min=0.5  stopband_max=1.0  filter_selection=1  gui_behaviour='Sysgen_GUI'  data_sign=Signed  data_width=16  data_fractional_bits=0  data_tuser_width=1  wrapper_available=true  ip_wrap_arbitrary_binary_point=true  ip_name=FIR Compiler  ip_version=7.2  dsptool_ready=true  ipcore_usecache=true  ipcore_useipmodelcache=true  port_translation_map={ 'aclken' => 'en', 'aresetn' => 'rst' }  run_core_at_system_period=true  ipcore_xco_need_fpga_part=true  block_type=fir_compiler_v7_2
      settings: infoedit=Maximum Possible : Maximizes oversampling rate. Abstracted input handshake (no s_data_tvalid) and automatic rate propagation.<br>Hardware Oversampling Rate : Specifies oversampling rate relative to the input sample period. Abstracted input handshake (no s_data_tvalid) and automatic rate propagation.<br>Input/Output Sample Period : Specifies absolute oversampling rate. No input handshake abstraction (exposes s_data_tvalid) and no rate propagation.
  FIR Stage 2 : xbsIndex_r4/FIR Compiler 7.2   Commented=on  coefficientvector=interpolation_single.getFilters.Stage2.Numerator/2  coefficient_sets=1  coefficient_reload=off  filter_type=Interpolation  rate_change_type=Integer  interpolation_rate=2  decimation_rate=1  zero_pack_factor=1  channel_sequence=Basic  number_channels=1  pattern_list='P4-0,P4-1,P4-2,P4-3,P4-4'  number_paths=1  ratespecification=Maximum_Possible  sampleperiod=0.25000000  hardwareoversamplingrate=1  coefficient_sign=Signed  quantization=Quantize_Only  coefficient_width=16  bestprecision=on  coefficient_fractional_bits=15  coefficient_structure=Inferred  output_rounding_mode=Full_Precision  output_width=31  filter_architecture=Systolic_Multiply_Accumulate  optimization_goal=Area  optimization_list='None'  data_buffer_type=Automatic  coefficient_buffer_type=Automatic  input_buffer_type=Automatic  output_buffer_type=Automatic  preference_for_other_storage=Automatic  multi_column_support=Automatic  columnconfig='4'  inter_column_pipe_length=4  data_has_tlast=Not_Required  m_data_has_tready=off  s_data_has_fifo=off  s_data_has_tuser=Not_Required  m_data_has_tuser=Not_Required  s_config_sync_mode=On_Vector  s_config_method=Single  num_reload_slots=1  has_aclken=off  has_aresetn=off  infoeditControl=ARESETn must be asserted for a minimum of 2 cycles  reset_data_vector=on  trim_axipin_name=on  simulation_type=hybrid_sim  simulation_model=sysgen:xfirv7_2_cmodel  data_path_portlist={ 's_axis_data_tdata', 'm_axis_data_tdata' }  passband_min=0.0  passband_max=0.5  stopband_min=0.5  stopband_max=1.0  filter_selection=1  gui_behaviour='Sysgen_GUI'  data_sign=Signed  data_width=16  data_fractional_bits=0  data_tuser_width=1  wrapper_available=true  ip_wrap_arbitrary_binary_point=true  ip_name=FIR Compiler  ip_version=7.2  dsptool_ready=true  ipcore_usecache=true  ipcore_useipmodelcache=true  port_translation_map={ 'aclken' => 'en', 'aresetn' => 'rst' }  run_core_at_system_period=true  ipcore_xco_need_fpga_part=true  block_type=fir_compiler_v7_2
      settings: infoedit=Maximum Possible : Maximizes oversampling rate. Abstracted input handshake (no s_data_tvalid) and automatic rate propagation.<br>Hardware Oversampling Rate : Specifies oversampling rate relative to the input sample period. Abstracted input handshake (no s_data_tvalid) and automatic rate propagation.<br>Input/Output Sample Period : Specifies absolute oversampling rate. No input handshake abstraction (exposes s_data_tvalid) and no rate propagation.
  FIR Stage 3 : xbsIndex_r4/FIR Compiler 7.2   Commented=on  coefficientvector=interpolation_single.getFilters.Stage3.Numerator/4  coefficient_sets=1  coefficient_reload=off  filter_type=Interpolation  rate_change_type=Integer  interpolation_rate=4  decimation_rate=1  zero_pack_factor=1  channel_sequence=Basic  number_channels=1  pattern_list='P4-0,P4-1,P4-2,P4-3,P4-4'  number_paths=1  ratespecification=Maximum_Possible  sampleperiod=0.25000000  hardwareoversamplingrate=1  coefficient_sign=Signed  quantization=Quantize_Only  coefficient_width=16  bestprecision=on  coefficient_fractional_bits=16  coefficient_structure=Inferred  output_rounding_mode=Full_Precision  output_width=31  filter_architecture=Systolic_Multiply_Accumulate  optimization_goal=Area  optimization_list='None'  data_buffer_type=Automatic  coefficient_buffer_type=Automatic  input_buffer_type=Automatic  output_buffer_type=Automatic  preference_for_other_storage=Automatic  multi_column_support=Automatic  columnconfig='5'  inter_column_pipe_length=4  data_has_tlast=Not_Required  m_data_has_tready=off  s_data_has_fifo=off  s_data_has_tuser=Not_Required  m_data_has_tuser=Not_Required  s_config_sync_mode=On_Vector  s_config_method=Single  num_reload_slots=1  has_aclken=off  has_aresetn=off  infoeditControl=ARESETn must be asserted for a minimum of 2 cycles  reset_data_vector=on  trim_axipin_name=on  simulation_type=hybrid_sim  simulation_model=sysgen:xfirv7_2_cmodel  data_path_portlist={ 's_axis_data_tdata', 'm_axis_data_tdata' }  passband_min=0.0  passband_max=0.5  stopband_min=0.5  stopband_max=1.0  filter_selection=1  gui_behaviour='Sysgen_GUI'  data_sign=Signed  data_width=16  data_fractional_bits=0  data_tuser_width=1  wrapper_available=true  ip_wrap_arbitrary_binary_point=true  ip_name=FIR Compiler  ip_version=7.2  dsptool_ready=true  ipcore_usecache=true  ipcore_useipmodelcache=true  port_translation_map={ 'aclken' => 'en', 'aresetn' => 'rst' }  run_core_at_system_period=true  ipcore_xco_need_fpga_part=true  block_type=fir_compiler_v7_2
      settings: infoedit=Maximum Possible : Maximizes oversampling rate. Abstracted input handshake (no s_data_tvalid) and automatic rate propagation.<br>Hardware Oversampling Rate : Specifies oversampling rate relative to the input sample period. Abstracted input handshake (no s_data_tvalid) and automatic rate propagation.<br>Input/Output Sample Period : Specifies absolute oversampling rate. No input handshake abstraction (exposes s_data_tvalid) and no rate propagation.
  FIR Stage 4 : xbsIndex_r4/FIR Compiler 7.2   Commented=on  coefficientvector=interpolation_single.getFilters.Stage4.Numerator/16  coefficient_sets=1  coefficient_reload=off  filter_type=Interpolation  rate_change_type=Integer  interpolation_rate=16  decimation_rate=1  zero_pack_factor=1  channel_sequence=Basic  number_channels=1  pattern_list='P4-0,P4-1,P4-2,P4-3,P4-4'  number_paths=1  ratespecification=Maximum_Possible  sampleperiod=0.25000000  hardwareoversamplingrate=1  coefficient_sign=Signed  quantization=Quantize_Only  coefficient_width=16  bestprecision=on  coefficient_fractional_bits=18  coefficient_structure=Inferred  output_rounding_mode=Full_Precision  output_width=31  filter_architecture=Systolic_Multiply_Accumulate  optimization_goal=Area  optimization_list='None'  data_buffer_type=Automatic  coefficient_buffer_type=Automatic  input_buffer_type=Automatic  output_buffer_type=Automatic  preference_for_other_storage=Automatic  multi_column_support=Automatic  columnconfig='4'  inter_column_pipe_length=4  data_has_tlast=Not_Required  m_data_has_tready=off  s_data_has_fifo=off  s_data_has_tuser=Not_Required  m_data_has_tuser=Not_Required  s_config_sync_mode=On_Vector  s_config_method=Single  num_reload_slots=1  has_aclken=off  has_aresetn=off  infoeditControl=ARESETn must be asserted for a minimum of 2 cycles  reset_data_vector=on  trim_axipin_name=on  simulation_type=hybrid_sim  simulation_model=sysgen:xfirv7_2_cmodel  data_path_portlist={ 's_axis_data_tdata', 'm_axis_data_tdata' }  passband_min=0.0  passband_max=0.5  stopband_min=0.5  stopband_max=1.0  filter_selection=1  gui_behaviour='Sysgen_GUI'  data_sign=Signed  data_width=16  data_fractional_bits=0  data_tuser_width=1  wrapper_available=true  ip_wrap_arbitrary_binary_point=true  ip_name=FIR Compiler  ip_version=7.2  dsptool_ready=true  ipcore_usecache=true  ipcore_useipmodelcache=true  port_translation_map={ 'aclken' => 'en', 'aresetn' => 'rst' }  run_core_at_system_period=true  ipcore_xco_need_fpga_part=true  block_type=fir_compiler_v7_2
      settings: infoedit=Maximum Possible : Maximizes oversampling rate. Abstracted input handshake (no s_data_tvalid) and automatic rate propagation.<br>Hardware Oversampling Rate : Specifies oversampling rate relative to the input sample period. Abstracted input handshake (no s_data_tvalid) and automatic rate propagation.<br>Input/Output Sample Period : Specifies absolute oversampling rate. No input handshake abstraction (exposes s_data_tvalid) and no rate propagation.
  Gateway Out : xbsIndex_r4/Gateway Out  inherit_from_input=on  hdl_port=off  rows=1  columns=1  UseAsDAC=off  DACChannel='1'  interface=None  automatic_assignment=on  address_offset=hex2dec('00')  intf_name=''  intf_description=''  timing_constraint=None  locs_specified=off  LOCs={}  io_standard={}  block_type=gatewayout
  Gateway Out1 : xbsIndex_r4/Gateway Out  inherit_from_input=on  hdl_port=off  rows=1  columns=1  UseAsDAC=off  DACChannel='1'  interface=None  automatic_assignment=on  address_offset=hex2dec('00')  intf_name=''  intf_description=''  timing_constraint=None  locs_specified=off  LOCs={}  io_standard={}  block_type=gatewayout
  Real-Imag to Complex : RealImagToComplex
  Spectrum Analyzer : SpectrumAnalyzer
  Terminator : Terminator
  Terminator{1..8} (8 alike) : Terminator  Commented=on
  Terminator9 : Terminator
  Real Out : Outport
  wires:
  FIR Stage 2/2 -> Terminator3/1
  FIR Stage 4/1 -> Terminator8/1
  ? -> Convert/1
  FIR Stage 2/1 -> Terminator4/1
  Convert2/1 -> FIR Stage 4/1
  ? -> Terminator2/1
  Convert3/1 -> Real Out/1
  Convert1/1 -> FIR Stage 3/1
  FIR Stage 4/2 -> Terminator7/1
  FIR Stage 4/3 -> Convert3/1
  Real In/1 -> FIR Stage 1/1
  Convert/1 -> FIR Stage 2/1
  FIR Stage 3/3 -> Convert2/1
  FIR Stage 3/2 -> Terminator5/1
  FIR Stage 3/1 -> Terminator6/1
  FIR Stage 2/3 -> Convert1/1
  ? -> Terminator1/1
  Imag In/1 -> FIR Stage 1/2
  FIR Stage 1/3 -> Convert4/1
  FIR Stage 1/4 -> Convert5/1
  Convert4/1 -> Gateway Out/1
  Convert5/1 -> Gateway Out1/1
  Gateway Out1/1 -> Real-Imag to Complex/2
  Gateway Out/1 -> Real-Imag to Complex/1
  Real-Imag to Complex/1 -> Spectrum Analyzer/1
  FIR Stage 1/2 -> Terminator/1
  FIR Stage 1/1 -> Terminator9/1

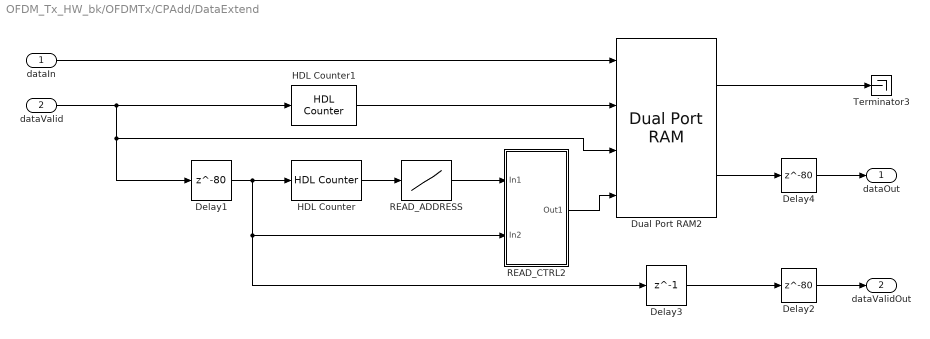
== system OFDM_Tx_HW_bk/OFDMTx/CPAdd/DataExtend ==
  dataIn : Inport
  dataValid : Inport  Port=2
  Delay1 : Delay  DelayLength=80  InitialCondition=0  UseCircularBuffer=on
  Delay2 : Delay  DelayLength=80
  Delay3 : Delay  DelayLength=1  InitialCondition=0  UseCircularBuffer=on
  Delay4 : Delay  DelayLength=80
  Dual Port RAM2 : hdlsllib/HDL RAMs/Dual Port RAM  ram_size=8
      settings: SourceProductBaseCode=SL
  HDL Counter : hdlsllib/Sources/HDL Counter  CountType=Count limited  CountInit=0  CountStep=1  CountMax=159  CountFromType=Initial value  CountFrom=0  CountResetPort=off  CountLoadPort=off  CountEnbPort=on  CountDirPort=off  CountDataType=Unsigned  CountWordLen=8  CountFracLen=0  CountSampTime=1
  HDL Counter1 : hdlsllib/Sources/HDL Counter  CountType=Count limited  CountInit=0  CountStep=1  CountMax=159  CountFromType=Initial value  CountFrom=0  CountResetPort=off  CountLoadPort=off  CountEnbPort=on  CountDirPort=off  CountDataType=Unsigned  CountWordLen=8  CountFracLen=0  CountSampTime=1
  READ_ADDRESS : Lookup_n-D  NumberOfTableDimensions=1  LookupTableObject=''  BreakpointsForDimension1=[0:159]  BreakpointsForDimension1FirstPoint=10  BreakpointsForDimension2FirstPoint=10  BreakpointsForDimension1Spacing=12  BreakpointsForDimension2Spacing=12  IndexSearchMethod=Evenly spaced points  Table=read_addr_cp  TableDataTypeStr=fixdt(0,8,0)  InterpMethod=Flat  DiagnosticForOutOfRangeInput=Error  InternalRulePriority=Speed  OutDataTypeStr=fixdt(0,8,0)  RndMeth=Simplest  InputSameDT=on
  READ_CTRL2 : Subsystem
  Terminator3 : Terminator
  dataOut : Outport  VectorParamsAs1DForOutWhenUnconnected=off
  dataValidOut : Outport  Port=2  VectorParamsAs1DForOutWhenUnconnected=off
  wires:
  Delay4/1 -> dataOut/1
  Delay2/1 -> dataValidOut/1
  Dual Port RAM2/1 -> Terminator3/1
  READ_ADDRESS/1 -> READ_CTRL2/1(In1)
  HDL Counter/1 -> READ_ADDRESS/1
  dataIn/1 -> Dual Port RAM2/1
  HDL Counter1/1 -> Dual Port RAM2/2
  Delay1/1 -> HDL Counter/1, Delay3/1, READ_CTRL2/2(In2)
  Dual Port RAM2/2 -> Delay4/1
  dataValid/1 -> HDL Counter1/1, Dual Port RAM2/3, Delay1/1
  Delay3/1 -> Delay2/1
  READ_CTRL2/1(Out1) -> Dual Port RAM2/4

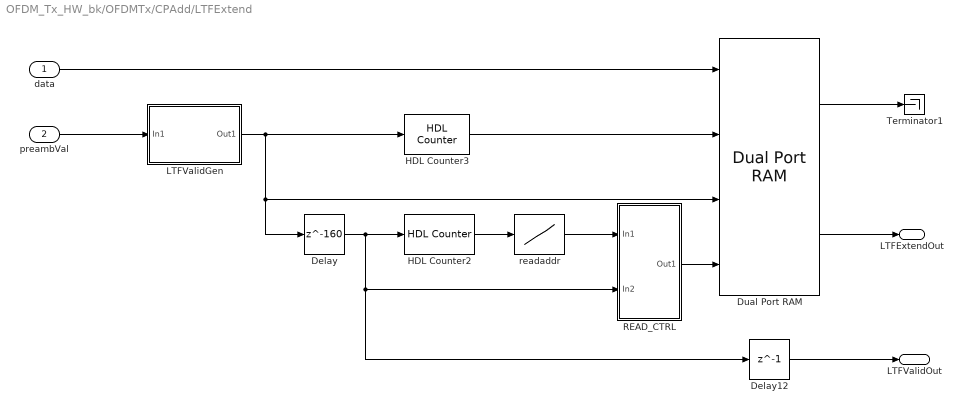
== system OFDM_Tx_HW_bk/OFDMTx/CPAdd/LTFExtend ==
  data : Inport
  preambVal : Inport  Port=2
  Delay : Delay  DelayLength=160  InitialCondition=0  UseCircularBuffer=on
  Delay12 : Delay  DelayLength=1  InitialCondition=0  UseCircularBuffer=on
  Dual Port RAM : hdlsllib/HDL RAMs/Dual Port RAM  ram_size=8
      settings: SourceProductBaseCode=SL
  HDL Counter2 : hdlsllib/Sources/HDL Counter  CountType=Count limited  CountInit=0  CountStep=1  CountMax=159  CountFromType=Initial value  CountFrom=0  CountResetPort=off  CountLoadPort=off  CountEnbPort=on  CountDirPort=off  CountDataType=Unsigned  CountWordLen=8  CountFracLen=0  CountSampTime=1
  HDL Counter3 : hdlsllib/Sources/HDL Counter  CountType=Count limited  CountInit=0  CountStep=1  CountMax=159  CountFromType=Initial value  CountFrom=0  CountResetPort=off  CountLoadPort=off  CountEnbPort=on  CountDirPort=off  CountDataType=Unsigned  CountWordLen=8  CountFracLen=0  CountSampTime=1
  LTFValidGen : Subsystem
  READ_CTRL : Subsystem
  Terminator1 : Terminator
  readaddr : Lookup_n-D  NumberOfTableDimensions=1  LookupTableObject=''  BreakpointsForDimension1=0:159  BreakpointsForDimension1FirstPoint=10  BreakpointsForDimension2FirstPoint=10  BreakpointsForDimension1Spacing=12  BreakpointsForDimension2Spacing=12  IndexSearchMethod=Evenly spaced points  Table=LTSread  TableDataTypeStr=fixdt(0,8,0)  InterpMethod=Flat  DiagnosticForOutOfRangeInput=Error  InternalRulePriority=Speed  OutDataTypeStr=fixdt(0,8,0)  RndMeth=Simplest  InputSameDT=on
  LTFExtendOut : Outport  VectorParamsAs1DForOutWhenUnconnected=off
  LTFValidOut : Outport  Port=2  VectorParamsAs1DForOutWhenUnconnected=off
  wires:
  readaddr/1 -> READ_CTRL/1(In1)
  READ_CTRL/1(Out1) -> Dual Port RAM/4
  HDL Counter3/1 -> Dual Port RAM/2
  Delay/1 -> READ_CTRL/2(In2), Delay12/1, HDL Counter2/1
  Dual Port RAM/1 -> Terminator1/1
  Delay12/1 -> LTFValidOut/1
  HDL Counter2/1 -> readaddr/1
  data/1 -> Dual Port RAM/1
  Dual Port RAM/2 -> LTFExtendOut/1
  preambVal/1 -> LTFValidGen/1(In1)
  LTFValidGen/1(Out1) -> Dual Port RAM/3, Delay/1, HDL Counter3/1

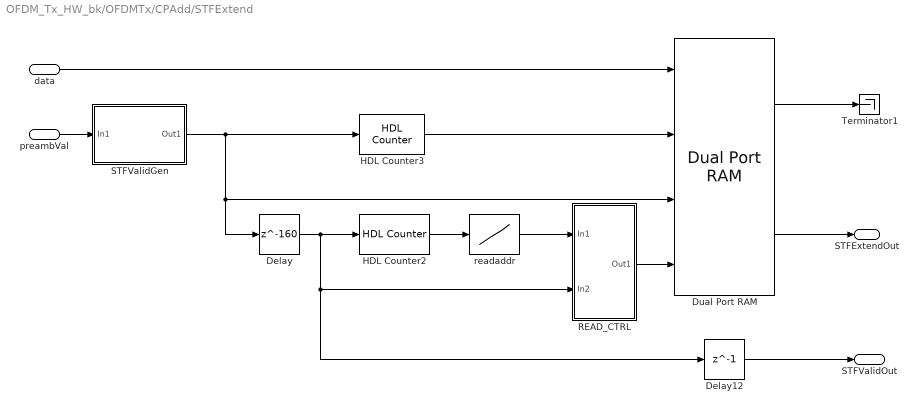
== system OFDM_Tx_HW_bk/OFDMTx/CPAdd/STFExtend ==
  data : Inport
  preambVal : Inport  Port=2
  Delay : Delay  DelayLength=160  InitialCondition=0  UseCircularBuffer=on
  Delay12 : Delay  DelayLength=1  InitialCondition=0  UseCircularBuffer=on
  Dual Port RAM : hdlsllib/HDL RAMs/Dual Port RAM  ram_size=8
      settings: SourceProductBaseCode=SL
  HDL Counter2 : hdlsllib/Sources/HDL Counter  CountType=Count limited  CountInit=0  CountStep=1  CountMax=159  CountFromType=Initial value  CountFrom=0  CountResetPort=off  CountLoadPort=off  CountEnbPort=on  CountDirPort=off  CountDataType=Unsigned  CountWordLen=8  CountFracLen=0  CountSampTime=1
  HDL Counter3 : hdlsllib/Sources/HDL Counter  CountType=Count limited  CountInit=0  CountStep=1  CountMax=159  CountFromType=Initial value  CountFrom=0  CountResetPort=off  CountLoadPort=off  CountEnbPort=on  CountDirPort=off  CountDataType=Unsigned  CountWordLen=8  CountFracLen=0  CountSampTime=1
  READ_CTRL : Subsystem
  STFValidGen : Subsystem
  Terminator1 : Terminator
  readaddr : Lookup_n-D  NumberOfTableDimensions=1  LookupTableObject=''  BreakpointsForDimension1=0:159  BreakpointsForDimension1FirstPoint=10  BreakpointsForDimension2FirstPoint=10  BreakpointsForDimension1Spacing=12  BreakpointsForDimension2Spacing=12  IndexSearchMethod=Evenly spaced points  Table=STSread  TableDataTypeStr=fixdt(0,8,0)  InterpMethod=Flat  DiagnosticForOutOfRangeInput=Error  InternalRulePriority=Speed  OutDataTypeStr=fixdt(0,8,0)  RndMeth=Simplest  InputSameDT=on
  STFExtendOut : Outport  VectorParamsAs1DForOutWhenUnconnected=off
  STFValidOut : Outport  Port=2  VectorParamsAs1DForOutWhenUnconnected=off
  wires:
  Dual Port RAM/2 -> STFExtendOut/1
  data/1 -> Dual Port RAM/1
  HDL Counter2/1 -> readaddr/1
  Delay12/1 -> STFValidOut/1
  Dual Port RAM/1 -> Terminator1/1
  Delay/1 -> HDL Counter2/1, Delay12/1, READ_CTRL/2(In2)
  HDL Counter3/1 -> Dual Port RAM/2
  READ_CTRL/1(Out1) -> Dual Port RAM/4
  preambVal/1 -> STFValidGen/1(In1)
  readaddr/1 -> READ_CTRL/1(In1)
  STFValidGen/1(Out1) -> HDL Counter3/1, Dual Port RAM/3, Delay/1

== system OFDM_Tx_HW_bk/OFDMTx/ControlSignalGenerator/PreamValidGen ==
  enable : Inport
  Compare To Constant : simulink/Logic and Bit Operations/Compare To Constant  relop===  const=320  OutDataTypeStr=boolean
  HDL Counter : hdlsllib/Sources/HDL Counter  CountType=Count limited  CountInit=0  CountStep=1  CountMax=320  CountFromType=Initial value  CountFrom=0  CountResetPort=on  CountLoadPort=off  CountEnbPort=on  CountDirPort=off  CountDataType=Unsigned  CountWordLen=9  CountFracLen=0  CountSampTime=1
  NOT : Logic  Operator=NOT  IconShape=distinctive  AllPortsSameDT=off  OutDataTypeStr=boolean
  RisingEdge : Subsystem
  Unit Delay Enabled Resettable Synchronous : hdlsllib/Discrete/Unit Delay Enabled Resettable Synchronous  InitialCondition=0.0  SampleTime=-1
      settings: SourceProductBaseCode=SL
  y : Outport  VectorParamsAs1DForOutWhenUnconnected=off
  wires:
  HDL Counter/1 -> Compare To Constant/1
  RisingEdge/1(Out1) -> Unit Delay Enabled Resettable Synchronous/2
  Compare To Constant/1 -> Unit Delay Enabled Resettable Synchronous/3
  enable/1 -> RisingEdge/1(In1), Unit Delay Enabled Resettable Synchronous/1, NOT/1, HDL Counter/2
  Unit Delay Enabled Resettable Synchronous/1 -> y/1
  NOT/1 -> HDL Counter/1

== system OFDM_Tx_HW_bk/OFDMTx/ControlSignalGenerator/dataReadyGen ==
  enb : Inport
  Compare To Constant : simulink/Logic and Bit Operations/Compare To Constant  relop=>  const=31  OutDataTypeStr=boolean
  HDL Counter : hdlsllib/Sources/HDL Counter  CountType=Count limited  CountInit=0  CountStep=1  CountMax=79  CountFromType=Initial value  CountFrom=0  CountResetPort=on  CountLoadPort=off  CountEnbPort=on  CountDirPort=off  CountDataType=Unsigned  CountWordLen=7  CountFracLen=0  CountSampTime=1
  NOT : Logic  Operator=NOT  IconShape=distinctive  AllPortsSameDT=off  OutDataTypeStr=boolean
  y : Outport
  wires:
  HDL Counter/1 -> Compare To Constant/1
  enb/1 -> NOT/1, HDL Counter/2
  NOT/1 -> HDL Counter/1
  Compare To Constant/1 -> y/1

== system OFDM_Tx_HW_bk/OFDMTx/ControlSignalGenerator/dataValidGen ==
  y : Inport
  enable : Inport  Port=2
  AND : Logic  IconShape=distinctive  AllPortsSameDT=off  OutDataTypeStr=boolean
  Delay : Delay  DelayLength=1
  NOT : Logic  Operator=NOT  IconShape=distinctive  AllPortsSameDT=off  OutDataTypeStr=boolean
  valOut : Outport
  wires:
  NOT/1 -> AND/1
  Delay/1 -> AND/2
  AND/1 -> valOut/1
  y/1 -> NOT/1
  enable/1 -> Delay/1
